simulink model "final_model"  (R2023b)
settings: Solver=VariableStepAuto  StartTime=0.0  StopTime=200  RelTol=1e-3
(part 1 of 3)
settings Model: Creator=Iustin  LastModifiedBy=Iustin

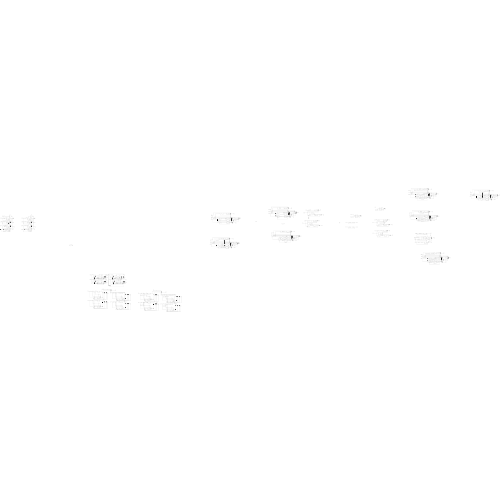
[thumbnail: Simulink's stored preview of the top-level diagram]
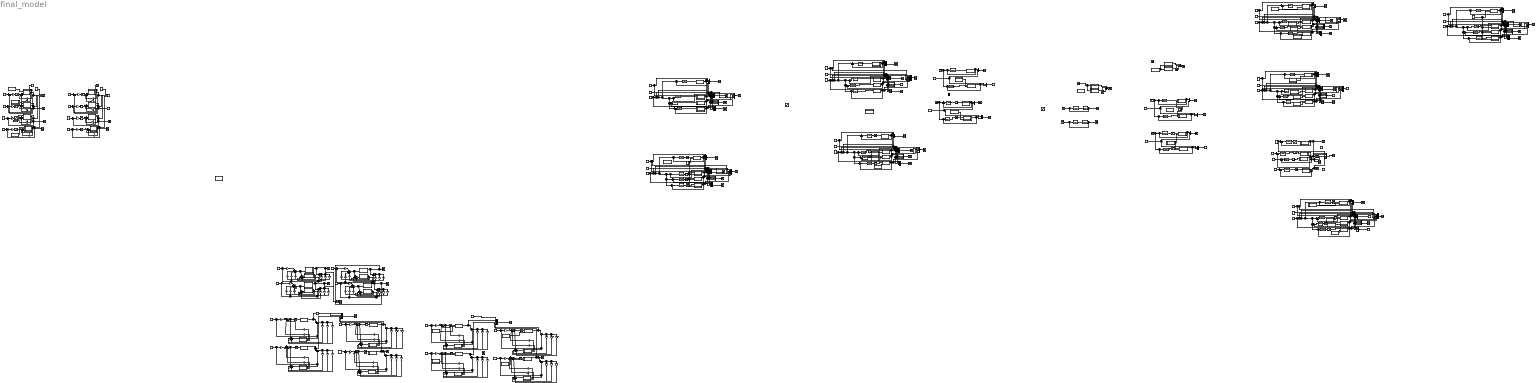
== system final_model ==
  "  G0 = 200" : Subsystem  mask{p1=0.005, p2=0.017, p3=0.00000808, n=0.175, V=120, Gb=80, G0=200}
  "  G0 = 4" : Subsystem  mask{p1=0.005, p2=0.017, p3=0.00000808, n=0.175, V=120, Gb=80, G0=200}
  " 100.1g" : Subsystem  mask{Gb=80, V=120, p1=0.032, p2=0.019, p3=0.00000987, n=0.208, G0=100}
  " 100.1g1" : Subsystem  mask{Gb=80, V=120, p1=0.032, p2=0.019, p3=0.00000987, n=0.208, G0=300}
  " G0 = 10" : Subsystem  mask{p1=0.005, p2=0.017, p3=0.00000808, n=0.175, V=120, Gb=80, G0=150}
  " G0 = 11" : Subsystem  mask{p1=0.005, p2=0.017, p3=0.00000808, n=0.175, V=120, Gb=80, G0=250}
  " G0 = 12" : Subsystem  mask{p1=0.005, p2=0.017, p3=0.00000808, n=0.175, V=120, Gb=80, G0=300}
  " G0 = 150" : Subsystem  mask{p1=0.005, p2=0.017, p3=0.00000808, n=0.175, V=120, Gb=80, G0=150}
  " G0 = 250" : Subsystem  mask{p1=0.005, p2=0.017, p3=0.00000808, n=0.175, V=120, Gb=80, G0=250}
  " G0 = 300" : Subsystem  mask{p1=0.005, p2=0.017, p3=0.00000808, n=0.175, V=120, Gb=80, G0=300}
  " Proces" : TransferFcn  Numerator=[-0.1741]  Denominator=[32320 6542 160.7 1]
  " Proces liniar" : Subsystem  mask{p1=0.005, p2=0.017, p3=0.00000808, n=0.175, V=120, Gb=80, G0=350, Xb=0.0054}
  " Proces liniar1" : Subsystem  mask{p1=0.005, p2=0.017, p3=0.00000808, n=0.175, V=120, Gb=80, G0=350, Xb=0.0054}
  " Proces liniar10" : Subsystem  mask{p1=0.005, p2=0.017, p3=0.00000808, n=0.175, V=120, Gb=80, G0=150, Xb=0.0054}
  " Proces liniar11" : Subsystem  mask{p1=0.005, p2=0.017, p3=0.00000808, n=0.175, V=120, Gb=80, G0=200, Xb=0.0054}
  " Proces liniar12" : Subsystem  mask{p1=0.005, p2=0.017, p3=0.00000808, n=0.175, V=120, Gb=80, G0=250, Xb=0.0054}
  " Proces liniar13" : Subsystem  mask{p1=0.005, p2=0.017, p3=0.00000808, n=0.175, V=120, Gb=80, G0=300, Xb=0.0054}
  " Proces liniar14" : Subsystem  mask{p1=0.005, p2=0.017, p3=0.00000808, n=0.175, V=120, Gb=80, G0=150, Xb=0.0054}
  " Proces liniar15" : Subsystem  mask{p1=0.005, p2=0.017, p3=0.00000808, n=0.175, V=120, Gb=80, G0=200, Xb=0.0054}
  " Proces liniar16" : Subsystem  mask{p1=0.005, p2=0.017, p3=0.00000808, n=0.175, V=120, Gb=80, G0=250, Xb=0.0054}
  " Proces liniar17" : Subsystem  mask{p1=0.005, p2=0.017, p3=0.00000808, n=0.175, V=120, Gb=80, G0=300, Xb=0.0054}
  " Proces liniar18" : Subsystem  mask{p1=0.005, p2=0.017, p3=0.00000808, n=0.175, V=120, Gb=80, G0=150, Xb=0.0054}
  " Proces liniar19" : Subsystem  mask{p1=0.005, p2=0.017, p3=0.00000808, n=0.175, V=120, Gb=80, G0=150, Xb=0.0054}
  " Proces liniar2" : Subsystem  mask{p1=0.005, p2=0.017, p3=0.00000808, n=0.175, V=120, Gb=80, G0=150, Xb=0.0054}
  " Proces liniar20" : Subsystem  mask{p1=0.005, p2=0.017, p3=0.00000808, n=0.175, V=120, Gb=80, G0=150, Xb=0.0054}
  " Proces liniar21" : Subsystem  mask{p1=0.005, p2=0.017, p3=0.00000808, n=0.175, V=120, Gb=80, G0=150, Xb=0.0054}
  " Proces liniar22" : Subsystem  mask{p1=0.005, p2=0.017, p3=0.00000808, n=0.175, V=120, Gb=80, G0=100, Xb=0.0054}
  " Proces liniar23" : Subsystem  mask{p1=0.005, p2=0.017, p3=0.00000808, n=0.175, V=120, Gb=80, G0=100, Xb=0.0054}
  " Proces liniar24" : Subsystem  mask{p1=0.005, p2=0.017, p3=0.00000808, n=0.175, V=120, Gb=80, G0=100, Xb=0.0054}
  " Proces liniar25" : Subsystem  mask{p1=0.005, p2=0.017, p3=0.00000808, n=0.175, V=120, Gb=80, G0=100, Xb=0.0054}
  " Proces liniar26" : Subsystem  mask{p1=0.005, p2=0.017, p3=0.00000808, n=0.175, V=120, Gb=80, G0=100, Xb=0.0054}
  " Proces liniar27" : Subsystem  mask{p1=0.005, p2=0.017, p3=0.00000808, n=0.175, V=120, Gb=80, G0=100, Xb=0.0054}
  " Proces liniar28" : Subsystem  mask{p1=0.005, p2=0.017, p3=0.00000808, n=0.175, V=120, Gb=80, G0=100, Xb=0.0054}
  " Proces liniar29" : Subsystem  mask{p1=0.005, p2=0.017, p3=0.00000808, n=0.175, V=120, Gb=80, G0=100, Xb=0.0054}
  " Proces liniar3" : Subsystem  mask{p1=0.005, p2=0.017, p3=0.00000808, n=0.175, V=120, Gb=80, G0=150, Xb=0.0054}
  " Proces liniar30" : Subsystem  mask{p1=0.005, p2=0.017, p3=0.00000808, n=0.175, V=120, Gb=80, G0=100, Xb=0.0054}
  " Proces liniar4" : Subsystem  mask{p1=0.005, p2=0.017, p3=0.00000808, n=0.175, V=120, Gb=80, G0=150, Xb=0.0054}
  " Proces liniar5" : Subsystem  mask{p1=0.005, p2=0.017, p3=0.00000808, n=0.175, V=120, Gb=80, G0=150, Xb=0.0054}
  " Proces liniar6" : Subsystem  mask{p1=0.005, p2=0.017, p3=0.00000808, n=0.175, V=120, Gb=80, G0=150, Xb=0.0054}
  " Proces liniar7" : Subsystem  mask{p1=0.005, p2=0.017, p3=0.00000808, n=0.175, V=120, Gb=80, G0=200, Xb=0.0054}
  " Proces liniar8" : Subsystem  mask{p1=0.005, p2=0.017, p3=0.00000808, n=0.175, V=120, Gb=80, G0=250, Xb=0.0054}
  " Proces liniar9" : Subsystem  mask{p1=0.005, p2=0.017, p3=0.00000808, n=0.175, V=120, Gb=80, G0=300, Xb=0.0054}
  " Proces neliniar" : Subsystem  mask{p1=0.005, p2=0.017, p3=0.00000808, n=0.175, V=120, Gb=80, G0=350}
  " Proces neliniar1" : Subsystem  mask{p1=0.005, p2=0.017, p3=0.00000808, n=0.175, V=120, Gb=80, G0=350}
  " Proces neliniar2" : Subsystem  mask{p1=0.005, p2=0.017, p3=0.00000808, n=0.175, V=120, Gb=80, G0=150}
  " Proces neliniar3" : Subsystem  mask{p1=0.005, p2=0.017, p3=0.00000808, n=0.175, V=120, Gb=80, G0=150}
  " Proces neliniar4" : Subsystem  mask{p1=0.005, p2=0.017, p3=0.00000808, n=0.175, V=120, Gb=80, G0=150}
  " Proces neliniar5" : Subsystem  mask{p1=0.005, p2=0.017, p3=0.00000808, n=0.175, V=120, Gb=80, G0=200}
  " Proces1" : TransferFcn  Numerator=[-0.1741]  Denominator=[32320 6542 160.7 1]
  " Regulator" : TransferFcn  Numerator=[-1454 -294.4 -7.231 -0.045]  Denominator=[171.2 34.28 1 0]
   Regulator plasar{,1..8,13..16} (13 alike) : TransferFcn  Numerator=[-1454 -294.4 -7.231 -0.045]  Denominator=[171.2 34.28 1 0]
  " Regulator plasare" : TransferFcn  Numerator=[-1454 -294.4 -7.231 -0.045]  Denominator=[171.2 34.28 1 0]
  " Regulator1" : TransferFcn  Numerator=[-1454 -294.4 -7.231 -0.045]  Denominator=[171.2 34.28 1 0]
   Regulator{2,4..6} (4 alike) : TransferFcn  Numerator=[-2843 -77.89 -0.5026]  Denominator=[0.5714 1 0]
  " Regulator3" : TransferFcn  Numerator=[-1454 -294.4 -7.231 -0.045]  Denominator=[171.2 34.28 1 0]
   RegulatorCMVK{,1..24} (25 alike) : TransferFcn  Numerator=[-2843 -77.89 -0.5026]  Denominator=[0.5714 1 0]
  10.1g : Subsystem  mask{Gb=80, V=120, p1=0.032, p2=0.019, p3=0.00000987, n=0.208, G0=100}
  10.1g1 : Subsystem  mask{Gb=80, V=120, p1=0.032, p2=0.019, p3=0.00000987, n=0.208, G0=150}
  1001g : Subsystem  mask{p1=0.005, p2=0.017, p3=0.00000808, n=0.175, V=120, Gb=80, G0=100}
  100g : Subsystem  mask{p1=0.005, p2=0.017, p3=0.00000808, n=0.175, V=120, Gb=80, G0=100}
  100g.1 : Subsystem  mask{p1=0.005, p2=0.017, p3=0.00000808, n=0.175, V=120, Gb=80, G0=100}
  10g : Subsystem  mask{p1=0.005, p2=0.017, p3=0.00000808, n=0.175, V=120, Gb=80, G0=100}
  10g.1 : Subsystem  mask{p1=0.005, p2=0.017, p3=0.00000808, n=0.175, V=120, Gb=80, G0=100}
  10g1 : Subsystem  mask{p1=0.005, p2=0.017, p3=0.00000808, n=0.175, V=120, Gb=80, G0=100}
  150gg : Subsystem  mask{p1=0.005, p2=0.017, p3=0.00000808, n=0.175, V=120, Gb=80, G0=150}
  200gg : Subsystem  mask{p1=0.005, p2=0.017, p3=0.00000808, n=0.175, V=120, Gb=80, G0=200}
  250gg : Subsystem  mask{p1=0.005, p2=0.017, p3=0.00000808, n=0.175, V=120, Gb=80, G0=250}
  300gg : Subsystem  mask{p1=0.005, p2=0.017, p3=0.00000808, n=0.175, V=120, Gb=80, G0=300}
  40.1g : Subsystem  mask{Gb=80, V=120, p1=0.032, p2=0.019, p3=0.00000987, n=0.208, G0=100}
  40.1g1 : Subsystem  mask{Gb=80, V=120, p1=0.032, p2=0.019, p3=0.00000987, n=0.208, G0=200}
  40g : Subsystem  mask{p1=0.005, p2=0.017, p3=0.00000808, n=0.175, V=120, Gb=80, G0=100}
  40g.1 : Subsystem  mask{p1=0.005, p2=0.017, p3=0.00000808, n=0.175, V=120, Gb=80, G0=100}
  40g1 : Subsystem  mask{p1=0.005, p2=0.017, p3=0.00000808, n=0.175, V=120, Gb=80, G0=100}
  70.1g : Subsystem  mask{Gb=80, V=120, p1=0.032, p2=0.019, p3=0.00000987, n=0.208, G0=100}
  70.1g1 : Subsystem  mask{Gb=80, V=120, p1=0.032, p2=0.019, p3=0.00000987, n=0.208, G0=250}
  70g : Subsystem  mask{p1=0.005, p2=0.017, p3=0.00000808, n=0.175, V=120, Gb=80, G0=100}
  70g.1 : Subsystem  mask{p1=0.005, p2=0.017, p3=0.00000808, n=0.175, V=120, Gb=80, G0=100}
  70g1 : Subsystem  mask{p1=0.005, p2=0.017, p3=0.00000808, n=0.175, V=120, Gb=80, G0=100}
  80 : Constant  Value=80
  Constant{,1..7,9,11..18,20..24,26..32} (29 alike) : Constant  Value=80
  Constant10 : Constant  Value=74
  Constant19 : Constant  Value=0
  Constant25 : Constant  Value=110
  Constant8 : Constant  Value=0
  DG 100g : Subsystem  mask{p1=0.005, p2=0.017, p3=0.00000808, n=0.175, V=120, Gb=80, G0=100}
  DG 10g : Subsystem  mask{p1=0.005, p2=0.017, p3=0.00000808, n=0.175, V=120, Gb=80, G0=100}
  DG 40g : Subsystem  mask{p1=0.005, p2=0.017, p3=0.00000808, n=0.175, V=120, Gb=80, G0=100}
  DG 70g : Subsystem  mask{p1=0.005, p2=0.017, p3=0.00000808, n=0.175, V=120, Gb=80, G0=100}
  K{1..3,10..13,25} (8 alike) : Gain  Gain=-10.1821
  K{4..6,14..15,17..18,36} (8 alike) : Gain  Gain=-1.4596e+05
  K{7..9,16,19..21,42} (8 alike) : Gain  Gain=0.0012
  K2.1 {,1..3} (4 alike) : Gain  Gain=-1.4472e+05
  K3.1 {,1..3} (4 alike) : Gain  Gain=-0.0018
  Ke1.{1..4} (4 alike) : Gain  Gain=-0.2134
  Ke2.{1..4} (4 alike) : Gain  Gain=0.0008
  Ke3.{1..4} (4 alike) : Gain  Gain=-8.4418
  Limita inferioara : Constant  Value=74
  Limita inferioara1 : Constant  Value=74
  Limita inferioara2 : Constant  Value=74
  Limita superioara : Constant  Value=110
  Limita superioara1 : Constant  Value=110
  Limita superioara2 : Constant  Value=110
  Maxim{1..5} (5 alike) : Constant  Value=110
  Minim{1..5} (5 alike) : Constant  Value=74
  Minim6 : Constant  Value=0
  Mux : Mux  Inputs=3
  Mux1 : Mux  Inputs=3
  Mux{3..10} (8 alike) : Mux  Inputs=2
  Mux11 : Mux  Inputs=7
  Mux{12..14,27,37,47,52..53} (8 alike) : Mux  Inputs=5
  Mux{15..26,28..31,33..36,38..41,43..46,48..51} (32 alike) : Mux
  Mux2 : Mux  Inputs=3
  Mux32 : Mux  Inputs=7
  Mux42 : Mux  Inputs=7
  Saturation : Saturate
  Saturation{1..12,14,18..22} (18 alike) : Saturate  UpperLimit=0  LowerLimit=-500
  Saturation{13,15..17,23..37} (19 alike) : Saturate  UpperLimit=500  LowerLimit=0
  Scope{,1..56,58..61,63..71,73..76} (74 alike) : Scope
  Scope57 : Scope  NumInputPorts=5
  Scope62 : Scope  NumInputPorts=5
  Scope72 : Scope  NumInputPorts=5
  Step{,1..9} (10 alike) : Step  SampleTime=0
  Sum{,1..46,48,50,52,54,57..58,62,64..65,68..70,73..74,77..78,81..82,85..86,89..90,93..94,97..98,101..102,104,106,108} (78 alike) : Sum  Inputs=|+-
  Sum{55..56,59..61,63,66..67,72,76,80,84,88,92,96,100} (16 alike) : Sum  Inputs=|++++
  Sum{47,49,51,53,103,105,107,109} (8 alike) : Sum  Inputs=|+++
  Sum{71,75,79,83,87,91,95,99} (8 alike) : Sum  Inputs=|+--
  Val. optima : Constant  Value=80
  Val. optima1 : Constant  Value=80
  Valoare optima{,1..7} (8 alike) : Constant  Value=80
  con : Constant  Value=80
  k{1,4,7,10,13..14,19,22} (8 alike) : Gain  Gain=-10.1821
  k1.1 {,1..3} (4 alike) : Gain  Gain=-45.1979
  k{2,5,8,11,15,17,20,23} (8 alike) : Gain  Gain=1.4596e+05
  k{3,6,9,12,16,18,21,24} (8 alike) : Gain  Gain=0.0012
  ke{1,4,7,10,13..14,19,22} (8 alike) : Gain  Gain=0.3304
  ke{2,5,8,11,15,17,20,23} (8 alike) : Gain  Gain=3.3886e-04
  ke{3,6,9,12,16,18,21,24} (8 alike) : Gain  Gain=0.1231
  kr.{1..4} (4 alike) : Gain  Gain=-9.1200e-04
  model liniar1 : Subsystem  mask{p1=0.032, p2=0.019, p3=0.00000987, V=120, Gb=80, Xb=0.0054, n=0.208, G0=150}
  model liniar2 : Subsystem  mask{p1=0.032, p2=0.019, p3=0.00000987, V=120, Gb=80, Xb=0.0054, n=0.208, G0=200}
  model liniar3 : Subsystem  mask{p1=0.032, p2=0.019, p3=0.00000987, V=120, Gb=80, Xb=0.0054, n=0.208, G0=250}
  model liniar4 : Subsystem  mask{p1=300, p2=0.019, p3=0.00000987, V=120, Gb=80, Xb=0.0054, n=0.208, G0=300}
  model_neliniar1 : Subsystem  mask{Gb=80, V=120, p1=0.032, p2=0.019, p3=0.00000987, n=0.208, G0=150}
  model_neliniar2 : Subsystem  mask{Gb=80, V=120, p1=0.032, p2=0.019, p3=0.00000987, n=0.208, G0=200}
  model_neliniar3 : Subsystem  mask{Gb=80, V=120, p1=0.032, p2=0.019, p3=0.00000987, n=0.208, G0=250}
  model_neliniar4 : Subsystem  mask{Gb=80, V=120, p1=0.032, p2=0.019, p3=0.00000987, n=0.208, G0=300}
  perturbatie1 : Subsystem  mask{Dg=100000, Ag=0.8, tg_max=40}
  perturbatie10 : Subsystem  mask{Dg=40*1000, Ag=0.8, tg_max=40}
  perturbatie11 : Subsystem  mask{Dg=100000, Ag=0.8, tg_max=40}
  perturbatie12 : Subsystem  mask{Dg=70*1000, Ag=0.8, tg_max=40}
  perturbatie13 : Subsystem  mask{Dg=100*1000, Ag=0.8, tg_max=40}
  perturbatie15 : Subsystem  mask{Dg=40*1000, Ag=0.8, tg_max=40}
  perturbatie16 : Subsystem  mask{Dg=70*1000, Ag=0.8, tg_max=40}
  perturbatie17 : Subsystem  mask{Dg=100*1000, Ag=0.8, tg_max=40}
  perturbatie18 : Subsystem  mask{Dg=10*1000, Ag=0.8, tg_max=40}
  perturbatie19 : Subsystem  mask{Dg=40, Ag=0.8, tg_max=40}
  perturbatie2 : Subsystem  mask{Dg=100000, Ag=0.8, tg_max=40}
  perturbatie20 : Subsystem  mask{Dg=70, Ag=0.8, tg_max=40}
  perturbatie21 : Subsystem  mask{Dg=100, Ag=0.8, tg_max=40}
  perturbatie22 : Subsystem  mask{Dg=10, Ag=0.8, tg_max=40}
  perturbatie23 : Subsystem  mask{Dg=40*1000, Ag=0.8, tg_max=40}
  perturbatie24 : Subsystem  mask{Dg=70*1000, Ag=0.8, tg_max=40}
  perturbatie25 : Subsystem  mask{Dg=100*1000, Ag=0.8, tg_max=40}
  perturbatie29 : Subsystem  mask{Dg=40*1000, Ag=0.8, tg_max=40}
  perturbatie3 : Subsystem  mask{Dg=10, Ag=0.8, tg_max=40}
  perturbatie30 : Subsystem  mask{Dg=70*1000, Ag=0.8, tg_max=40}
  perturbatie31 : Subsystem  mask{Dg=100*1000, Ag=0.8, tg_max=40}
  perturbatie36 : Subsystem  mask{Dg=10*1000, Ag=0.8, tg_max=40}
  perturbatie37 : Subsystem  mask{Dg=40*1000, Ag=0.8, tg_max=40}
  perturbatie38 : Subsystem  mask{Dg=70*1000, Ag=0.8, tg_max=40}
  perturbatie39 : Subsystem  mask{Dg=100*1000, Ag=0.8, tg_max=40}
  perturbatie4 : Subsystem  mask{Dg=10, Ag=0.8, tg_max=40}
  perturbatie5 : Subsystem  mask{Dg=10, Ag=0.8, tg_max=40}
  perturbatie6 : Subsystem  mask{Dg=30, Ag=0.8, tg_max=40}
  perturbatie7 : Subsystem  mask{Dg=40*1000, Ag=0.8, tg_max=40}
  perturbatie8 : Subsystem  mask{Dg=10*1000, Ag=0.8, tg_max=40}
  perturbatie9 : Subsystem  mask{Dg=10*1000, Ag=0.8, tg_max=40}
  wires:
  " Proces liniar"/1(" G(t)") -> Mux/1
  " Proces neliniar"/1(" G(t)") -> Mux/2
  Step/1 -> Mux/3
  Mux/1 -> Scope/1
  perturbatie1/1(p(t)) -> " Proces liniar"/2(p(t)), " Proces neliniar"/2(p(t))
  Mux1/1 -> Scope1/1
  Step2/1 -> Mux1/3
  " Proces neliniar1"/1(" G(t)") -> Mux1/2
  " Proces liniar1"/1(" G(t)") -> Mux1/1
  Step3/1 -> " Proces neliniar1"/1(" u(t)"), " Proces liniar1"/1(" u(t)")
  Sum/1 -> " Regulator"/1
  " Regulator"/1 -> " Proces"/1
  Step6/1 -> Sum2/1, Sum1/1
  Sum1/1 -> " Regulator1"/1
  " Regulator1"/1 -> Saturation2/1
  " Proces neliniar2"/1(" G(t)") -> Sum2/2, Mux3/1
  " Proces liniar2"/1(" G(t)") -> Mux4/1, Sum1/2
  Sum2/1 -> " Regulator plasare"/1
  " Regulator plasare"/1 -> Saturation1/1
  Saturation1/1 -> " Proces neliniar2"/1(" u(t)")
  Mux3/1 -> Scope4/1
  Constant/1 -> Mux4/2, Mux3/2
  Mux4/1 -> Scope3/1
  Saturation2/1 -> " Proces liniar2"/1(" u(t)")
  " Proces"/1 -> Scope2/1, Sum/2
  " Regulator3"/1 -> " Proces liniar3"/1(" u(t)")
  " Proces neliniar3"/1(" G(t)") -> Sum4/2, Mux6/1
  Mux6/1 -> Scope6/1
  Mux7/1 -> Scope5/1
  " Regulator plasar"/1 -> " Proces neliniar3"/1(" u(t)")
  Constant3/1 -> Mux7/2, Mux6/2
  Sum3/1 -> " Regulator3"/1
  " Proces liniar3"/1(" G(t)") -> Mux7/1, Sum3/2
  Step5/1 -> Sum4/1, Sum3/1
  perturbatie4/1(p(t)) -> " Proces neliniar3"/2(p(t))
  Sum4/1 -> " Regulator plasar"/1
  Step4/1 -> Sum/1
  Sum5/1 -> " Regulator5"/1
  " Regulator5"/1 -> " Proces1"/1
  " Proces1"/1 -> Scope7/1, Sum5/2
  Step7/1 -> Sum5/1
  " Proces liniar4"/1(" G(t)") -> Mux8/1, Sum6/2
  Constant1/1 -> Mux8/2, Mux5/2
  " Regulator4"/1 -> " Proces liniar4"/1(" u(t)")
  " Regulator2"/1 -> " Proces neliniar4"/1(" u(t)")
  Mux8/1 -> Scope8/1
  Mux5/1 -> Scope9/1
  Step8/1 -> Sum7/1, Sum6/1
  " Proces neliniar4"/1(" G(t)") -> Sum7/2, Mux5/1
  Sum7/1 -> " Regulator2"/1
  Sum6/1 -> " Regulator4"/1
  " Regulator6"/1 -> Saturation5/1
  " Proces neliniar5"/1(" G(t)") -> Sum9/2, Mux9/1
  Mux9/1 -> Scope11/1
  Saturation5/1 -> " Proces neliniar5"/1(" u(t)")
  Saturation6/1 -> " Proces liniar5"/1(" u(t)")
  Step9/1 -> Sum9/1, Sum8/1
  Mux10/1 -> Scope10/1
  Constant2/1 -> Mux10/2, Mux9/2
  Sum8/1 -> " RegulatorCMVK"/1
  " RegulatorCMVK"/1 -> Saturation6/1
  " Proces liniar5"/1(" G(t)") -> Mux10/1, Sum8/2
  Sum9/1 -> " Regulator6"/1
  perturbatie6/1(p(t)) -> " Proces neliniar5"/2(p(t)), " Proces liniar5"/2(p(t))
  perturbatie3/1(p(t)) -> " Proces neliniar2"/2(p(t))
  Sum10/1 -> " Regulator plasar1"/1
  Sum11/1 -> " Regulator plasar2"/1
  Sum12/1 -> " Regulator plasar3"/1
  Sum13/1 -> " Regulator plasar4"/1
  Mux11/1 -> Scope16/1
  Constant19/1 -> " Proces neliniar4"/2(p(t)), " Proces liniar4"/2(p(t))
  Sum22/1 -> " RegulatorCMVK5"/1
  Sum23/1 -> " RegulatorCMVK6"/1
  Constant23/1 -> Sum24/1
  Constant24/1 -> Sum25/1
  10g/1(" G(t)") -> Sum22/2, Mux14/1, Scope27/1
  " RegulatorCMVK5"/1 -> Saturation9/1
  Mux14/1 -> Scope31/1
  80/1 -> Mux14/5, Sum22/1
  " RegulatorCMVK6"/1 -> Saturation10/1
  70g/1(" G(t)") -> Scope29/1, Mux14/3, Sum24/2
  Sum24/1 -> " RegulatorCMVK7"/1
  100g/1(" G(t)") -> Mux14/4, Scope28/1, Sum25/2
  40g/1(" G(t)") -> Mux14/2, Scope30/1, Sum23/2
  con/1 -> Sum23/1
  Sum25/1 -> " RegulatorCMVK8"/1
  " RegulatorCMVK7"/1 -> Saturation11/1
  Saturation9/1 -> 10g/1(" u(t)")
  Saturation10/1 -> 40g/1(" u(t)")
  Saturation11/1 -> 70g/1(" u(t)")
  " RegulatorCMVK8"/1 -> Saturation12/1
  Saturation12/1 -> 100g/1(" u(t)")
  Mux16/1 -> Scope12/1
  Valoare optima/1 -> Mux19/4, Mux18/4, Mux17/4, Mux11/5, Mux16/4, Sum10/1, Sum13/1, Sum12/1, Sum11/1
  " G0 = 300"/1(" G(t)") -> Mux11/4, Mux19/1, Sum13/2
  Mux19/1 -> Scope13/1
  "  G0 = 200"/1(" G(t)") -> Mux11/2, Mux17/1, Sum11/2
  Mux17/1 -> Scope15/1
  Mux18/1 -> Scope14/1
  " G0 = 150"/1(" G(t)") -> Sum10/2, Mux11/1, Mux16/1
  Limita inferioara/1 -> Mux19/2, Mux18/2, Mux17/2, Mux11/7, Mux16/2
  Limita superioara/1 -> Mux11/6, Mux19/3, Mux18/3, Mux17/3, Mux16/3
  " G0 = 250"/1(" G(t)") -> Mux11/3, Mux18/1, Sum12/2
  DG 40g/1(" G(t)") -> Mux12/2, Mux21/1, Sum15/2
  DG 70g/1(" G(t)") -> Mux12/3, Mux22/1, Sum16/2
  Minim1/1 -> Mux23/2, Mux22/2, Mux21/2, Mux20/2
  Mux22/1 -> Scope19/1
  Mux21/1 -> Scope20/1
  Mux20/1 -> Scope17/1
  DG 10g/1(" G(t)") -> Sum14/2, Mux12/1, Mux20/1
  Maxim1/1 -> Mux20/3, Mux23/3, Mux22/3, Mux21/3
  Valoare optima1/1 -> Mux23/4, Mux22/4, Mux21/4, Mux12/5, Mux20/4, Sum14/1, Sum17/1, Sum16/1, Sum15/1
  Mux12/1 -> Scope21/1
  Sum16/1 -> " Regulator plasar7"/1
  DG 100g/1(" G(t)") -> Mux12/4, Mux23/1, Sum17/2
  Sum15/1 -> " Regulator plasar6"/1
  Sum17/1 -> " Regulator plasar8"/1
  Sum14/1 -> " Regulator plasar5"/1
  Mux23/1 -> Scope18/1
  " Regulator plasar5"/1 -> Saturation22/1
  " Regulator plasar6"/1 -> Saturation4/1
  " Regulator plasar7"/1 -> Saturation7/1
  40g1/1(" G(t)") -> Mux13/2, Mux24/1, Sum19/2
  " RegulatorCMVK2"/1 -> 40g1/1(" u(t)")
  70g1/1(" G(t)") -> Mux13/3, Mux25/1, Sum20/2
  Minim2/1 -> Mux26/2, Mux25/2, Mux24/2, Mux15/2
  Mux25/1 -> Scope24/1
  " RegulatorCMVK3"/1 -> 70g1/1(" u(t)")
  Mux24/1 -> Scope25/1
  Mux15/1 -> Scope22/1
  " RegulatorCMVK4"/1 -> 1001g/1(" u(t)")
  10g1/1(" G(t)") -> Sum18/2, Mux13/1, Mux15/1
  Maxim2/1 -> Mux15/3, Mux26/3, Mux25/3, Mux24/3
  Valoare optima2/1 -> Mux26/4, Mux25/4, Mux24/4, Mux13/5, Mux15/4, Sum18/1, Sum21/1, Sum20/1, Sum19/1
  Mux13/1 -> Scope26/1
  Sum20/1 -> " RegulatorCMVK3"/1
  1001g/1(" G(t)") -> Mux13/4, Mux26/1, Sum21/2
  Sum19/1 -> " RegulatorCMVK2"/1
  Sum21/1 -> " RegulatorCMVK4"/1
  Sum18/1 -> " RegulatorCMVK1"/1
  Mux26/1 -> Scope23/1
  " RegulatorCMVK1"/1 -> 10g1/1(" u(t)")
  " Proces liniar6"/1(" G(t)") -> Sum26/2, Mux27/1, Mux28/1
  " RegulatorCMVK20"/1 -> " Proces liniar9"/1(" u(t)")
  Mux31/1 -> Scope33/1
  Maxim3/1 -> Mux31/3, Mux30/3, Mux29/3, Mux28/3
  Minim3/1 -> Mux31/2, Mux30/2, Mux29/2, Mux28/2
  Sum27/1 -> " RegulatorCMVK18"/1
  Mux30/1 -> Scope34/1
  " RegulatorCMVK19"/1 -> " Proces liniar8"/1(" u(t)")
  " Proces liniar7"/1(" G(t)") -> Mux27/2, Mux29/1, Sum27/2
  Valoare optima3/1 -> Mux31/4, Mux30/4, Mux29/4, Mux27/5, Mux28/4, Sum26/1, Sum29/1, Sum28/1, Sum27/1
  " Proces liniar9"/1(" G(t)") -> Mux27/4, Mux31/1, Sum29/2
  Mux28/1 -> Scope32/1
  Mux27/1 -> Scope36/1
  " RegulatorCMVK17"/1 -> " Proces liniar6"/1(" u(t)")
  Sum29/1 -> " RegulatorCMVK20"/1
  " Proces liniar8"/1(" G(t)") -> Mux27/3, Mux30/1, Sum28/2
  Sum28/1 -> " RegulatorCMVK19"/1
  " RegulatorCMVK18"/1 -> " Proces liniar7"/1(" u(t)")
  Mux29/1 -> Scope35/1
  Sum26/1 -> " RegulatorCMVK17"/1
  Sum30/1 -> " Regulator plasar16"/1
  " Regulator plasar13"/1 -> Saturation15/1
  " Proces liniar13"/1(" G(t)") -> Mux32/4, Mux36/1, Sum33/2
  Sum32/1 -> " Regulator plasar14"/1
  " Proces liniar11"/1(" G(t)") -> Mux32/2, Mux34/1, Sum31/2
  " Regulator plasar16"/1 -> Saturation14/1
  Mux34/1 -> Scope40/1
  Constant8/1 -> " Proces liniar10"/2(p(t)), " Proces liniar11"/2(p(t)), " Proces liniar13"/2(p(t)), " Proces liniar12"/2(p(t))
  Sum33/1 -> " Regulator plasar15"/1
  " Proces liniar12"/1(" G(t)") -> Mux32/3, Mux35/1, Sum32/2
  Mux32/1 -> Scope41/1
  Mux33/1 -> Scope37/1
  " Regulator plasar14"/1 -> Saturation16/1
  Sum31/1 -> " Regulator plasar13"/1
  Mux35/1 -> Scope39/1
  Maxim4/1 -> Mux32/7, Mux36/3, Mux35/3, Mux34/3, Mux33/3
  Minim4/1 -> Mux36/2, Mux35/2, Mux34/2, Mux32/6, Mux33/2
  " Regulator plasar15"/1 -> Saturation17/1
  Valoare optima4/1 -> Mux36/4, Mux35/4, Mux34/4, Mux32/5, Mux33/4, Sum30/1, Sum33/1, Sum32/1, Sum31/1
  Mux36/1 -> Scope38/1
  " Proces liniar10"/1(" G(t)") -> Sum30/2, Mux32/1, Mux33/1
  Saturation14/1 -> " Proces liniar10"/1(" u(t)")
  Saturation15/1 -> " Proces liniar11"/1(" u(t)")
  Saturation16/1 -> " Proces liniar12"/1(" u(t)")
  Saturation17/1 -> " Proces liniar13"/1(" u(t)")
  perturbatie18/1(p(t)) -> " Proces liniar18"/2(p(t))
  perturbatie15/1(p(t)) -> " Proces liniar19"/2(p(t))
  perturbatie16/1(p(t)) -> " Proces liniar20"/2(p(t))
  Mux41/1 -> Scope43/1
  Limita superioara1/1 -> Mux41/3, Mux40/3, Mux39/3, Mux38/3
  " Proces liniar18"/1(" G(t)") -> Sum34/2, Mux37/1, Mux38/1
  " RegulatorCMVK9"/1 -> " Proces liniar18"/1(" u(t)")
  Mux40/1 -> Scope44/1
  " Proces liniar20"/1(" G(t)") -> Mux37/3, Mux40/1, Sum36/2
  Limita inferioara1/1 -> Mux41/2, Mux40/2, Mux39/2, Mux38/2
  Mux39/1 -> Scope45/1
  " Proces liniar19"/1(" G(t)") -> Mux37/2, Mux39/1, Sum35/2
  Mux38/1 -> Scope42/1
  Valoare optima5/1 -> Mux41/4, Mux40/4, Mux39/4, Mux37/5, Mux38/4, Sum34/1, Sum37/1, Sum36/1, Sum35/1
  Sum37/1 -> " RegulatorCMVK11"/1
  Mux37/1 -> Scope46/1
  Sum34/1 -> " RegulatorCMVK9"/1
  Sum36/1 -> " RegulatorCMVK12"/1
  Sum35/1 -> " RegulatorCMVK10"/1
  " RegulatorCMVK10"/1 -> " Proces liniar19"/1(" u(t)")
  " RegulatorCMVK12"/1 -> " Proces liniar20"/1(" u(t)")
  " RegulatorCMVK13"/1 -> Saturation19/1
  Sum41/1 -> " RegulatorCMVK14"/1
  Sum39/1 -> " RegulatorCMVK13"/1
  " G0 = 10"/1(" G(t)") -> Sum38/2, Mux42/1, Mux43/1
  Sum38/1 -> " RegulatorCMVK16"/1
  " RegulatorCMVK16"/1 -> Saturation18/1
  Limita inferioara2/1 -> Mux46/2, Mux45/2, Mux44/2, Mux42/7, Mux43/2
  "  G0 = 4"/1(" G(t)") -> Mux42/2, Mux44/1, Sum39/2
  Mux43/1 -> Scope47/1
  perturbatie19/1(p(t)) -> "  G0 = 4"/2(p(t))
  perturbatie22/1(p(t)) -> " G0 = 10"/2(p(t))
  Limita superioara2/1 -> Mux42/6, Mux46/3, Mux45/3, Mux44/3, Mux43/3
  Mux46/1 -> Scope48/1
  Mux42/1 -> Scope51/1
  Valoare optima6/1 -> Mux46/4, Mux45/4, Mux44/4, Mux42/5, Mux43/4, Sum38/1, Sum41/1, Sum40/1, Sum39/1
  " G0 = 12"/1(" G(t)") -> Mux42/4, Mux46/1, Sum41/2
  Mux44/1 -> Scope50/1
  perturbatie20/1(p(t)) -> " G0 = 11"/2(p(t))
  perturbatie21/1(p(t)) -> " G0 = 12"/2(p(t))
  " G0 = 11"/1(" G(t)") -> Mux42/3, Mux45/1, Sum40/2
  " RegulatorCMVK14"/1 -> Saturation21/1
  Sum40/1 -> " RegulatorCMVK15"/1
  Mux45/1 -> Scope49/1
  Saturation18/1 -> " G0 = 10"/1(" u(t)")
  Saturation19/1 -> "  G0 = 4"/1(" u(t)")
  " RegulatorCMVK15"/1 -> Saturation20/1
  Saturation20/1 -> " G0 = 11"/1(" u(t)")
  Saturation21/1 -> " G0 = 12"/1(" u(t)")
  " Regulator plasar1"/1 -> " G0 = 150"/1(" u(t)")
  " Regulator plasar2"/1 -> "  G0 = 200"/1(" u(t)")
  " Regulator plasar3"/1 -> " G0 = 250"/1(" u(t)")
  " Regulator plasar4"/1 -> " G0 = 300"/1(" u(t)")
  Saturation22/1 -> DG 10g/1(" u(t)")
  Saturation4/1 -> DG 40g/1(" u(t)")
  Saturation7/1 -> DG 70g/1(" u(t)")
  " Regulator plasar8"/1 -> Saturation8/1
  Saturation8/1 -> DG 100g/1(" u(t)")
  perturbatie23/1(p(t)) -> DG 40g/2(p(t))
  perturbatie24/1(p(t)) -> DG 70g/2(p(t))
  perturbatie25/1(p(t)) -> DG 100g/2(p(t))
  perturbatie9/1(p(t)) -> 10g1/2(p(t))
  perturbatie29/1(p(t)) -> 40g1/2(p(t))
  perturbatie30/1(p(t)) -> 70g1/2(p(t))
  perturbatie31/1(p(t)) -> 1001g/2(p(t))
  Sum43/1 -> " RegulatorCMVK22"/1
  " RegulatorCMVK22"/1 -> " Proces liniar15"/1(" u(t)")
  Sum44/1 -> " RegulatorCMVK23"/1
  Sum42/1 -> " RegulatorCMVK21"/1
  Minim5/1 -> Mux51/2, Mux50/2, Mux49/2, Mux48/2
  Mux48/1 -> Scope52/1
  " RegulatorCMVK24"/1 -> " Proces liniar17"/1(" u(t)")
  Maxim5/1 -> Mux51/3, Mux50/3, Mux49/3, Mux48/3
  " Proces liniar15"/1(" G(t)") -> Mux47/2, Mux49/1, Sum43/2
  Mux50/1 -> Scope54/1
  " Proces liniar16"/1(" G(t)") -> Mux47/3, Mux50/1, Sum44/2
  Mux47/1 -> Scope56/1
  Valoare optima7/1 -> Mux51/4, Mux50/4, Mux49/4, Mux47/5, Mux48/4, Sum42/1, Sum45/1, Sum44/1, Sum43/1
  " Proces liniar17"/1(" G(t)") -> Mux47/4, Mux51/1, Sum45/2
  " Proces liniar14"/1(" G(t)") -> Sum42/2, Mux47/1, Mux48/1
  " RegulatorCMVK21"/1 -> " Proces liniar14"/1(" u(t)")
  Mux51/1 -> Scope53/1
  Mux49/1 -> Scope55/1
  Sum45/1 -> " RegulatorCMVK24"/1
  " RegulatorCMVK23"/1 -> " Proces liniar16"/1(" u(t)")
  Minim6/1 -> " Proces liniar15"/2(p(t)), " Proces liniar16"/2(p(t)), " Proces liniar17"/2(p(t)), " Proces liniar14"/2(p(t))
  " RegulatorCMVK11"/1 -> " Proces liniar21"/1(" u(t)")
  perturbatie17/1(p(t)) -> " Proces liniar21"/2(p(t))
  " Proces liniar21"/1(" G(t)") -> Sum37/2, Mux37/4, Mux41/1
  Val. optima/1 -> Scope57/1
  " 100.1g"/1(G(t)) -> Scope61/1, Scope57/5, Sum52/2
  40.1g/1(G(t)) -> Scope57/3, Scope59/1, Sum48/2
  Sum48/1 -> K1/1
  Sum50/1 -> K2/1
  70.1g/2(X(t)) -> K5/1
  10.1g/3(I(t)) -> K42/1
  Constant12/1 -> Sum50/1
  10.1g/1(G(t)) -> Sum46/2, Scope57/2, Scope58/1
  40.1g/3(I(t)) -> K7/1
  " 100.1g"/3(I(t)) -> K9/1
  K8/1 -> Sum51/3
  K5/1 -> Sum51/2
  K7/1 -> Sum49/3
  Sum53/1 -> " 100.1g"/2(u(t))
  40.1g/2(X(t)) -> K4/1
  K6/1 -> Sum53/2
  K4/1 -> Sum49/2
  70.1g/3(I(t)) -> K8/1
  70.1g/1(G(t)) -> Scope57/4, Scope60/1, Sum50/2
  " 100.1g"/2(X(t)) -> K6/1
  Sum52/1 -> K3/1
  Constant11/1 -> Sum48/1
  Constant4/1 -> Sum46/1
  Constant13/1 -> Sum52/1
  Sum49/1 -> 40.1g/2(u(t))
  K9/1 -> Sum53/3
  Sum46/1 -> K25/1
  Sum51/1 -> 70.1g/2(u(t))
  K42/1 -> Sum47/3
  10.1g/2(X(t)) -> K36/1
  K36/1 -> Sum47/2
  Sum47/1 -> 10.1g/2(u(t))
  perturbatie36/1(p(t)) -> 10.1g/1(p(t))
  perturbatie37/1(p(t)) -> 40.1g/1(p(t))
  perturbatie38/1(p(t)) -> 70.1g/1(p(t))
  perturbatie39/1(p(t)) -> " 100.1g"/1(p(t))
  K25/1 -> Saturation23/1
  Saturation23/1 -> Sum47/1
  K1/1 -> Saturation13/1
  Saturation13/1 -> Sum49/1
  K2/1 -> Saturation24/1
  Saturation24/1 -> Sum51/1
  K3/1 -> Saturation25/1
  Saturation25/1 -> Sum53/1
  model liniar3/1(G(t)) -> K3.1 2/1
  K3.1 3/1 -> Sum55/4
  Ke2.4/1 -> Sum56/3
  Ke3.1/1 -> Sum61/2
  Sum60/1 -> model_neliniar1/2(u(t)), Sum61/1
  Sum59/1 -> Sum63/1, model_neliniar2/2(u(t))
  kr.4/1 -> Sum55/1
  Constant9/1 -> Sum65/1
  Sum56/1 -> model liniar4/2(u(t))
  K2.1 3/1 -> Sum55/2
  Ke2.1/1 -> Sum61/3
  Sum57/1 -> Ke1.4/1, Ke2.4/1, Ke3.4/1
  model_neliniar3/1(G(t)) -> Sum68/1, Scope62/4, Scope64/1
  Sum62/1 -> Ke1.1/1, Ke2.1/1, Ke3.1/1
  model liniar3/2(X(t)) -> K2.1 2/1
  Sum64/1 -> Ke1.2/1, Ke2.2/1, Ke3.2/1
  Sum63/1 -> model liniar2/2(u(t))
  model liniar2/2(X(t)) -> K2.1 1/1
  Ke3.2/1 -> Sum63/2
  model liniar1/3(I(t)) -> Sum62/2, Sum58/2, "k1.1 "/1
  "K3.1 "/1 -> Sum60/4
  kr.2/1 -> Sum59/1
  Ke1.2/1 -> Sum63/4
  k1.1 1/1 -> Sum59/3
  Sum54/1 -> kr.2/1
  model liniar2/1(G(t)) -> K3.1 1/1
  Constant5/1 -> Scope62/1
  Sum61/1 -> model liniar1/2(u(t))
  Sum58/1 -> kr.1/1
  "K2.1 "/1 -> Sum60/2
  Ke1.1/1 -> Sum61/4
  kr.3/1 -> Sum66/1
  Ke2.2/1 -> Sum63/3
  K2.1 1/1 -> Sum59/2
  model liniar4/1(G(t)) -> K3.1 3/1
  model liniar4/2(X(t)) -> K2.1 3/1
  K3.1 2/1 -> Sum66/4
  k1.1 2/1 -> Sum66/3
  model_neliniar4/1(G(t)) -> Sum57/1, Scope65/1, Scope62/5
  Ke1.3/1 -> Sum67/4
  kr.1/1 -> Sum60/1
  model liniar1/1(G(t)) -> "K3.1 "/1
  k1.1 3/1 -> Sum55/3
  Sum68/1 -> Ke1.3/1, Ke2.3/1, Ke3.3/1
  Ke3.4/1 -> Sum56/2
  Sum67/1 -> model liniar3/2(u(t))
  model_neliniar1/1(G(t)) -> Sum62/1, Scope62/2, Scope66/1
  model_neliniar2/1(G(t)) -> Sum64/1, Scope62/3, Scope63/1
  model liniar3/3(I(t)) -> Sum68/2, Sum65/2, k1.1 2/1
  Constant6/1 -> Sum58/1
  Ke1.4/1 -> Sum56/4
  Ke3.3/1 -> Sum67/2
  model liniar2/3(I(t)) -> Sum64/2, Sum54/2, k1.1 1/1
  model liniar1/2(X(t)) -> "K2.1 "/1
  "k1.1 "/1 -> Sum60/3
  model liniar4/3(I(t)) -> Sum57/2, Sum69/2, k1.1 3/1
  Ke2.3/1 -> Sum67/3
  Constant7/1 -> Sum54/1
  Sum66/1 -> model_neliniar3/2(u(t)), Sum67/1
  Constant14/1 -> Sum69/1
  Sum69/1 -> kr.4/1
  Sum65/1 -> kr.3/1
  Sum55/1 -> model_neliniar4/2(u(t)), Sum56/1
  K3.1 1/1 -> Sum59/4
  K2.1 2/1 -> Sum66/2
  Constant15/1 -> Sum70/1
  Sum70/1 -> k1/1
  k1/1 -> Sum71/1
  Sum71/1 -> Saturation26/1, Sum72/1
  Sum72/1 -> " Proces liniar23"/1(" u(t)")
  150gg/1(" G(t)") -> Mux52/1, Sum73/1
  Sum73/1 -> ke1/1, ke2/1, ke3/1
  ke1/1 -> Sum72/2
  ke2/1 -> Sum72/3
  ke3/1 -> Sum72/4
  " Proces liniar23"/3(I(t)) -> k3/1
  " Proces liniar23"/2(X(t)) -> k2/1
  " Proces liniar23"/1(" G(t)") -> Sum70/2, Sum73/2
  k2/1 -> Sum71/3
  k3/1 -> Sum71/2
  Mux52/1 -> Scope67/1
  Constant16/1 -> Mux52/2
  Saturation26/1 -> 150gg/1(" u(t)")
  200gg/1(" G(t)") -> Mux52/3, Sum77/1
  k4/1 -> Sum75/1
  Saturation27/1 -> 200gg/1(" u(t)")
  ke5/1 -> Sum76/3
  Sum77/1 -> ke4/1, ke5/1, ke6/1
  " Proces liniar24"/3(I(t)) -> k6/1
  k5/1 -> Sum75/2
  " Proces liniar24"/2(X(t)) -> k5/1
  Constant17/1 -> Sum74/1
  Sum76/1 -> " Proces liniar24"/1(" u(t)")
  ke4/1 -> Sum76/2
  ke6/1 -> Sum76/4
  Sum74/1 -> k4/1
  Sum75/1 -> Saturation27/1, Sum76/1
  " Proces liniar24"/1(" G(t)") -> Sum74/2, Sum77/2
  k6/1 -> Sum75/3
  250gg/1(" G(t)") -> Mux52/4, Sum81/1
  k7/1 -> Sum79/1
  Saturation28/1 -> 250gg/1(" u(t)")
  ke8/1 -> Sum80/3
  Sum81/1 -> ke7/1, ke8/1, ke9/1
  " Proces liniar25"/3(I(t)) -> k9/1
  k8/1 -> Sum79/2
  " Proces liniar25"/2(X(t)) -> k8/1
  Constant20/1 -> Sum78/1
  Sum80/1 -> " Proces liniar25"/1(" u(t)")
  ke7/1 -> Sum80/2
  ke9/1 -> Sum80/4
  Sum78/1 -> k7/1
  Sum79/1 -> Saturation28/1, Sum80/1
  " Proces liniar25"/1(" G(t)") -> Sum78/2, Sum81/2
  k9/1 -> Sum79/3
  k10/1 -> Sum83/1
  Saturation29/1 -> 300gg/1(" u(t)")
  ke11/1 -> Sum84/3
  Sum85/1 -> ke10/1, ke11/1, ke12/1
  " Proces liniar26"/3(I(t)) -> k12/1
  k11/1 -> Sum83/2
  " Proces liniar26"/2(X(t)) -> k11/1
  Constant22/1 -> Sum82/1
  Sum84/1 -> " Proces liniar26"/1(" u(t)")
  ke10/1 -> Sum84/2
  ke12/1 -> Sum84/4
  Sum82/1 -> k10/1
  Sum83/1 -> Saturation29/1, Sum84/1
  " Proces liniar26"/1(" G(t)") -> Sum82/2, Sum85/2
  k12/1 -> Sum83/3
  300gg/1(" G(t)") -> Mux52/5, Scope68/1, Sum85/1
  Sum95/1 -> Saturation32/1, Sum96/1
  k16/1 -> Sum99/3
  k15/1 -> Sum99/2
  Sum99/1 -> Saturation33/1, Sum100/1
  k18/1 -> Sum87/2
  k23/1 -> Sum95/2
  k19/1 -> Sum91/1
  k21/1 -> Sum91/3
  " Proces liniar30"/2(X(t)) -> k15/1
  k22/1 -> Sum95/1
  Sum88/1 -> " Proces liniar27"/1(" u(t)")
  100g.1/1(" G(t)") -> Mux53/5, Scope70/1, Sum101/1
  Sum97/1 -> ke22/1, ke23/1, ke24/1
  ke14/1 -> Sum100/2
  k14/1 -> Sum99/1
  Sum98/1 -> k14/1
  Sum87/1 -> Saturation30/1, Sum88/1
  k20/1 -> Sum91/2
  k24/1 -> Sum95/3
  Sum89/1 -> ke13/1, ke17/1, ke18/1
  " Proces liniar30"/1(" G(t)") -> Sum98/2, Sum101/2
  Mux53/1 -> Scope69/1
  Saturation30/1 -> 10g.1/1(" u(t)")
  Sum100/1 -> " Proces liniar30"/1(" u(t)")
  ke18/1 -> Sum88/4
  Constant28/1 -> Sum98/1
  " Proces liniar30"/3(I(t)) -> k16/1
  ke24/1 -> Sum96/4
  ke15/1 -> Sum100/3
  " Proces liniar28"/2(X(t)) -> k20/1
  Sum94/1 -> k22/1
  ke16/1 -> Sum100/4
  Sum101/1 -> ke14/1, ke15/1, ke16/1
  " Proces liniar29"/1(" G(t)") -> Sum94/2, Sum97/2
  k17/1 -> Sum87/3
  Saturation33/1 -> 100g.1/1(" u(t)")
  Constant21/1 -> Mux53/2
  Sum91/1 -> Saturation31/1, Sum92/1
  Constant26/1 -> Sum90/1
  Sum96/1 -> " Proces liniar29"/1(" u(t)")
  " Proces liniar27"/3(I(t)) -> k18/1
  " Proces liniar29"/3(I(t)) -> k24/1
  " Proces liniar29"/2(X(t)) -> k23/1
  Constant27/1 -> Sum94/1
  ke23/1 -> Sum96/3
  ke17/1 -> Sum88/3
  Sum92/1 -> " Proces liniar28"/1(" u(t)")
  Sum86/1 -> k13/1
  10g.1/1(" G(t)") -> Mux53/1, Sum89/1
  " Proces liniar27"/1(" G(t)") -> Sum86/2, Sum89/2
  Saturation32/1 -> 70g.1/1(" u(t)")
  Sum90/1 -> k19/1
  70g.1/1(" G(t)") -> Mux53/4, Sum97/1
  ke22/1 -> Sum96/2
  ke20/1 -> Sum92/3
  " Proces liniar28"/1(" G(t)") -> Sum90/2, Sum93/2
  40g.1/1(" G(t)") -> Mux53/3, Sum93/1
  ke21/1 -> Sum92/4
  k13/1 -> Sum87/1
  ke13/1 -> Sum88/2
  ke19/1 -> Sum92/2
  Constant18/1 -> Sum86/1
  " Proces liniar28"/3(I(t)) -> k21/1
  Saturation31/1 -> 40g.1/1(" u(t)")
  Sum93/1 -> ke19/1, ke20/1, ke21/1
  " Proces liniar27"/2(X(t)) -> k17/1
  perturbatie8/1(p(t)) -> 10g.1/2(p(t))
  perturbatie10/1(p(t)) -> 40g.1/2(p(t))
  perturbatie12/1(p(t)) -> 70g.1/2(p(t))
  perturbatie13/1(p(t)) -> 100g.1/2(p(t))
  Sum104/1 -> K10/1
  Sum105/1 -> 40.1g1/2(u(t))
  70.1g1/2(X(t)) -> K17/1
  K15/1 -> Sum105/2
  Saturation35/1 -> Sum103/1
  Sum102/1 -> K12/1
  K13/1 -> Saturation37/1
  K19/1 -> Sum105/3
  K21/1 -> Sum109/3
  Constant31/1 -> Sum108/1
  K17/1 -> Sum107/2
  10.1g1/1(G(t)) -> Sum102/2, Scope72/2, Scope73/1
  K10/1 -> Saturation34/1
  Val. optima1/1 -> Scope72/1
  K12/1 -> Saturation35/1
  Saturation36/1 -> Sum107/1
  Sum108/1 -> K13/1
  K20/1 -> Sum107/3
  Saturation37/1 -> Sum109/1
  K11/1 -> Saturation36/1
  Sum103/1 -> 10.1g1/2(u(t))
  40.1g1/1(G(t)) -> Scope72/3, Scope74/1, Sum104/2
  K18/1 -> Sum109/2
  40.1g1/3(I(t)) -> K19/1
  Sum109/1 -> " 100.1g1"/2(u(t))
  40.1g1/2(X(t)) -> K15/1
  10.1g1/3(I(t)) -> K16/1
  Constant32/1 -> Sum102/1
  K16/1 -> Sum103/3
  70.1g1/1(G(t)) -> Scope72/4, Scope75/1, Sum106/2
  Constant30/1 -> Sum106/1
  " 100.1g1"/1(G(t)) -> Scope76/1, Scope72/5, Sum108/2
  70.1g1/3(I(t)) -> K20/1
  K14/1 -> Sum103/2
  Sum106/1 -> K11/1
  " 100.1g1"/2(X(t)) -> K18/1
  " 100.1g1"/3(I(t)) -> K21/1
  Constant29/1 -> Sum104/1
  Saturation34/1 -> Sum105/1
  10.1g1/2(X(t)) -> K14/1
  Sum107/1 -> 70.1g1/2(u(t))

== system final_model/  G0 = 200 ==
  " u(t)" : Inport
  p(t) : Inport  Port=2
  Constant : Constant  Value=p1*Gb
  Constant1 : Constant  Value=p1
  Gain : Gain  Gain=1/V
  Gain1 : Gain  Gain=n
  Gain2 : Gain  Gain=p3
  Gain3 : Gain  Gain=-p2
  Gain4 : Gain  Gain=1/V
  Integrator : Integrator
  Integrator1 : Integrator
  Integrator2 : Integrator  InitialCondition=G0
  Product : Product
  Sum : Sum  Inputs=|+-
  Sum1 : Sum  Inputs=|++
  Sum2 : Sum  Inputs=|++-
  Sum3 : Sum  Inputs=|++
  " G(t)" : Outport
  X(t) : Outport  Port=2
  I(t) : Outport  Port=3
  wires:
  " u(t)"/1 -> Gain/1
  Gain/1 -> Sum/1
  Sum/1 -> Integrator/1
  Integrator/1 -> Gain2/1, I(t)/1, Gain1/1
  Gain1/1 -> Sum/2
  Gain2/1 -> Sum1/1
  Gain3/1 -> Sum1/2
  Integrator1/1 -> Gain3/1, Sum3/2, X(t)/1
  p(t)/1 -> Gain4/1
  Gain4/1 -> Sum2/1
  Constant/1 -> Sum2/2
  Constant1/1 -> Sum3/1
  Sum2/1 -> Integrator2/1
  Product/1 -> Sum2/3
  Sum3/1 -> Product/2
  Integrator2/1 -> Product/1, " G(t)"/1
  Sum1/1 -> Integrator1/1

== system final_model/  G0 = 4 ==
  " u(t)" : Inport
  p(t) : Inport  Port=2
  Constant : Constant  Value=p1*Gb
  Constant1 : Constant  Value=p1
  Gain : Gain  Gain=1/V
  Gain1 : Gain  Gain=n
  Gain2 : Gain  Gain=p3
  Gain3 : Gain  Gain=-p2
  Gain4 : Gain  Gain=1/V
  Integrator : Integrator
  Integrator1 : Integrator
  Integrator2 : Integrator  InitialCondition=G0
  Product : Product
  Sum : Sum  Inputs=|+-
  Sum1 : Sum  Inputs=|++
  Sum2 : Sum  Inputs=|++-
  Sum3 : Sum  Inputs=|++
  " G(t)" : Outport
  X(t) : Outport  Port=2
  I(t) : Outport  Port=3
  wires:
  " u(t)"/1 -> Gain/1
  Gain/1 -> Sum/1
  Sum/1 -> Integrator/1
  Integrator/1 -> Gain2/1, I(t)/1, Gain1/1
  Gain1/1 -> Sum/2
  Gain2/1 -> Sum1/1
  Gain3/1 -> Sum1/2
  Integrator1/1 -> Gain3/1, Sum3/2, X(t)/1
  p(t)/1 -> Gain4/1
  Gain4/1 -> Sum2/1
  Constant/1 -> Sum2/2
  Constant1/1 -> Sum3/1
  Sum2/1 -> Integrator2/1
  Product/1 -> Sum2/3
  Sum3/1 -> Product/2
  Integrator2/1 -> Product/1, " G(t)"/1
  Sum1/1 -> Integrator1/1

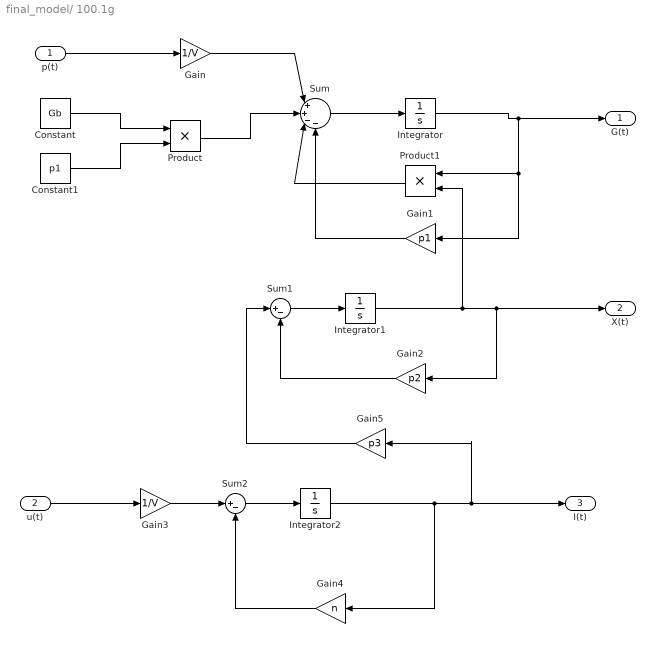
== system final_model/ 100.1g ==
  p(t) : Inport
  u(t) : Inport  Port=2
  Constant : Constant  Value=Gb
  Constant1 : Constant  Value=p1
  Gain : Gain  Gain=1/V
  Gain1 : Gain  Gain=p1
  Gain2 : Gain  Gain=p2
  Gain3 : Gain  Gain=1/V
  Gain4 : Gain  Gain=n
  Gain5 : Gain  Gain=p3
  Integrator : Integrator  InitialCondition=G0
  Integrator1 : Integrator
  Integrator2 : Integrator
  Product : Product
  Product1 : Product
  Sum : Sum  Inputs=|++--
  Sum1 : Sum  Inputs=|+-
  Sum2 : Sum  Inputs=|+-
  G(t) : Outport
  X(t) : Outport  Port=2
  I(t) : Outport  Port=3
  wires:
  Sum2/1 -> Integrator2/1
  Gain3/1 -> Sum2/1
  Sum1/1 -> Integrator1/1
  Integrator2/1 -> Gain4/1, I(t)/1, Gain5/1
  u(t)/1 -> Gain3/1
  Integrator1/1 -> Product1/2, X(t)/1, Gain2/1
  Product/1 -> Sum/2
  Integrator/1 -> G(t)/1, Gain1/1, Product1/1
  Gain5/1 -> Sum1/1
  Sum/1 -> Integrator/1
  Constant1/1 -> Product/2
  Constant/1 -> Product/1
  Gain4/1 -> Sum2/2
  Gain2/1 -> Sum1/2
  Product1/1 -> Sum/3
  Gain1/1 -> Sum/4
  p(t)/1 -> Gain/1
  Gain/1 -> Sum/1

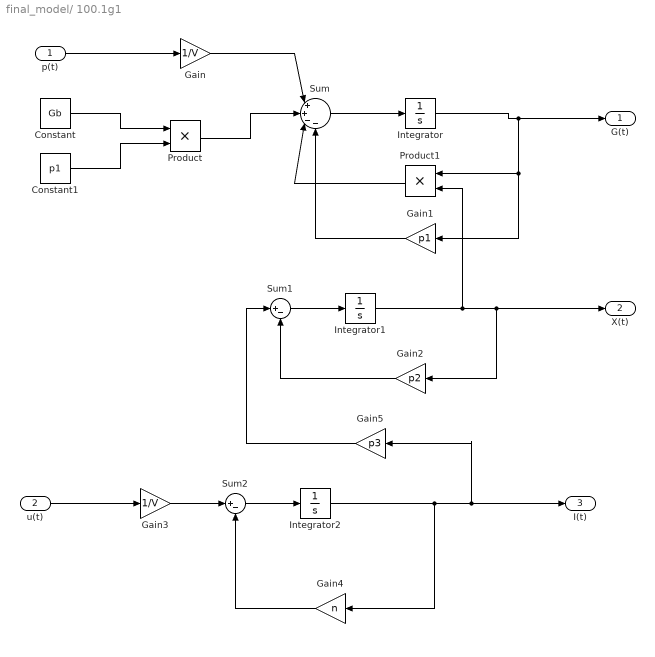
== system final_model/ 100.1g1 ==
  p(t) : Inport
  u(t) : Inport  Port=2
  Constant : Constant  Value=Gb
  Constant1 : Constant  Value=p1
  Gain : Gain  Gain=1/V
  Gain1 : Gain  Gain=p1
  Gain2 : Gain  Gain=p2
  Gain3 : Gain  Gain=1/V
  Gain4 : Gain  Gain=n
  Gain5 : Gain  Gain=p3
  Integrator : Integrator  InitialCondition=G0
  Integrator1 : Integrator
  Integrator2 : Integrator
  Product : Product
  Product1 : Product
  Sum : Sum  Inputs=|++--
  Sum1 : Sum  Inputs=|+-
  Sum2 : Sum  Inputs=|+-
  G(t) : Outport
  X(t) : Outport  Port=2
  I(t) : Outport  Port=3
  wires:
  Sum2/1 -> Integrator2/1
  Gain3/1 -> Sum2/1
  Sum1/1 -> Integrator1/1
  Integrator2/1 -> Gain4/1, I(t)/1, Gain5/1
  u(t)/1 -> Gain3/1
  Integrator1/1 -> Product1/2, X(t)/1, Gain2/1
  Product/1 -> Sum/2
  Integrator/1 -> G(t)/1, Gain1/1, Product1/1
  Gain5/1 -> Sum1/1
  Sum/1 -> Integrator/1
  Constant1/1 -> Product/2
  Constant/1 -> Product/1
  Gain4/1 -> Sum2/2
  Gain2/1 -> Sum1/2
  Product1/1 -> Sum/3
  Gain1/1 -> Sum/4
  p(t)/1 -> Gain/1
  Gain/1 -> Sum/1

== system final_model/ G0 = 10 ==
  " u(t)" : Inport
  p(t) : Inport  Port=2
  Constant : Constant  Value=p1*Gb
  Constant1 : Constant  Value=p1
  Gain : Gain  Gain=1/V
  Gain1 : Gain  Gain=n
  Gain2 : Gain  Gain=p3
  Gain3 : Gain  Gain=-p2
  Gain4 : Gain  Gain=1/V
  Integrator : Integrator
  Integrator1 : Integrator
  Integrator2 : Integrator  InitialCondition=G0
  Product : Product
  Sum : Sum  Inputs=|+-
  Sum1 : Sum  Inputs=|++
  Sum2 : Sum  Inputs=|++-
  Sum3 : Sum  Inputs=|++
  " G(t)" : Outport
  X(t) : Outport  Port=2
  I(t) : Outport  Port=3
  wires:
  " u(t)"/1 -> Gain/1
  Gain/1 -> Sum/1
  Sum/1 -> Integrator/1
  Integrator/1 -> Gain2/1, I(t)/1, Gain1/1
  Gain1/1 -> Sum/2
  Gain2/1 -> Sum1/1
  Gain3/1 -> Sum1/2
  Integrator1/1 -> Gain3/1, Sum3/2, X(t)/1
  p(t)/1 -> Gain4/1
  Gain4/1 -> Sum2/1
  Constant/1 -> Sum2/2
  Constant1/1 -> Sum3/1
  Sum2/1 -> Integrator2/1
  Product/1 -> Sum2/3
  Sum3/1 -> Product/2
  Integrator2/1 -> Product/1, " G(t)"/1
  Sum1/1 -> Integrator1/1

== system final_model/ G0 = 11 ==
  " u(t)" : Inport
  p(t) : Inport  Port=2
  Constant : Constant  Value=p1*Gb
  Constant1 : Constant  Value=p1
  Gain : Gain  Gain=1/V
  Gain1 : Gain  Gain=n
  Gain2 : Gain  Gain=p3
  Gain3 : Gain  Gain=-p2
  Gain4 : Gain  Gain=1/V
  Integrator : Integrator
  Integrator1 : Integrator
  Integrator2 : Integrator  InitialCondition=G0
  Product : Product
  Sum : Sum  Inputs=|+-
  Sum1 : Sum  Inputs=|++
  Sum2 : Sum  Inputs=|++-
  Sum3 : Sum  Inputs=|++
  " G(t)" : Outport
  X(t) : Outport  Port=2
  I(t) : Outport  Port=3
  wires:
  " u(t)"/1 -> Gain/1
  Gain/1 -> Sum/1
  Sum/1 -> Integrator/1
  Integrator/1 -> Gain2/1, I(t)/1, Gain1/1
  Gain1/1 -> Sum/2
  Gain2/1 -> Sum1/1
  Gain3/1 -> Sum1/2
  Integrator1/1 -> Gain3/1, Sum3/2, X(t)/1
  p(t)/1 -> Gain4/1
  Gain4/1 -> Sum2/1
  Constant/1 -> Sum2/2
  Constant1/1 -> Sum3/1
  Sum2/1 -> Integrator2/1
  Product/1 -> Sum2/3
  Sum3/1 -> Product/2
  Integrator2/1 -> Product/1, " G(t)"/1
  Sum1/1 -> Integrator1/1

== system final_model/ G0 = 12 ==
  " u(t)" : Inport
  p(t) : Inport  Port=2
  Constant : Constant  Value=p1*Gb
  Constant1 : Constant  Value=p1
  Gain : Gain  Gain=1/V
  Gain1 : Gain  Gain=n
  Gain2 : Gain  Gain=p3
  Gain3 : Gain  Gain=-p2
  Gain4 : Gain  Gain=1/V
  Integrator : Integrator
  Integrator1 : Integrator
  Integrator2 : Integrator  InitialCondition=G0
  Product : Product
  Sum : Sum  Inputs=|+-
  Sum1 : Sum  Inputs=|++
  Sum2 : Sum  Inputs=|++-
  Sum3 : Sum  Inputs=|++
  " G(t)" : Outport
  X(t) : Outport  Port=2
  I(t) : Outport  Port=3
  wires:
  " u(t)"/1 -> Gain/1
  Gain/1 -> Sum/1
  Sum/1 -> Integrator/1
  Integrator/1 -> Gain2/1, I(t)/1, Gain1/1
  Gain1/1 -> Sum/2
  Gain2/1 -> Sum1/1
  Gain3/1 -> Sum1/2
  Integrator1/1 -> Gain3/1, Sum3/2, X(t)/1
  p(t)/1 -> Gain4/1
  Gain4/1 -> Sum2/1
  Constant/1 -> Sum2/2
  Constant1/1 -> Sum3/1
  Sum2/1 -> Integrator2/1
  Product/1 -> Sum2/3
  Sum3/1 -> Product/2
  Integrator2/1 -> Product/1, " G(t)"/1
  Sum1/1 -> Integrator1/1

== system final_model/ G0 = 150 ==
  " u(t)" : Inport
  p(t) : Inport  Port=2
  Constant : Constant  Value=p1*Gb
  Constant1 : Constant  Value=p1
  Gain : Gain  Gain=1/V
  Gain1 : Gain  Gain=n
  Gain2 : Gain  Gain=p3
  Gain3 : Gain  Gain=-p2
  Gain4 : Gain  Gain=1/V
  Integrator : Integrator
  Integrator1 : Integrator
  Integrator2 : Integrator  InitialCondition=G0
  Product : Product
  Sum : Sum  Inputs=|+-
  Sum1 : Sum  Inputs=|++
  Sum2 : Sum  Inputs=|++-
  Sum3 : Sum  Inputs=|++
  " G(t)" : Outport
  X(t) : Outport  Port=2
  I(t) : Outport  Port=3
  wires:
  " u(t)"/1 -> Gain/1
  Gain/1 -> Sum/1
  Sum/1 -> Integrator/1
  Integrator/1 -> Gain2/1, I(t)/1, Gain1/1
  Gain1/1 -> Sum/2
  Gain2/1 -> Sum1/1
  Gain3/1 -> Sum1/2
  Integrator1/1 -> Gain3/1, Sum3/2, X(t)/1
  p(t)/1 -> Gain4/1
  Gain4/1 -> Sum2/1
  Constant/1 -> Sum2/2
  Constant1/1 -> Sum3/1
  Sum2/1 -> Integrator2/1
  Product/1 -> Sum2/3
  Sum3/1 -> Product/2
  Integrator2/1 -> Product/1, " G(t)"/1
  Sum1/1 -> Integrator1/1

== system final_model/ G0 = 250 ==
  " u(t)" : Inport
  p(t) : Inport  Port=2
  Constant : Constant  Value=p1*Gb
  Constant1 : Constant  Value=p1
  Gain : Gain  Gain=1/V
  Gain1 : Gain  Gain=n
  Gain2 : Gain  Gain=p3
  Gain3 : Gain  Gain=-p2
  Gain4 : Gain  Gain=1/V
  Integrator : Integrator
  Integrator1 : Integrator
  Integrator2 : Integrator  InitialCondition=G0
  Product : Product
  Sum : Sum  Inputs=|+-
  Sum1 : Sum  Inputs=|++
  Sum2 : Sum  Inputs=|++-
  Sum3 : Sum  Inputs=|++
  " G(t)" : Outport
  X(t) : Outport  Port=2
  I(t) : Outport  Port=3
  wires:
  " u(t)"/1 -> Gain/1
  Gain/1 -> Sum/1
  Sum/1 -> Integrator/1
  Integrator/1 -> Gain2/1, I(t)/1, Gain1/1
  Gain1/1 -> Sum/2
  Gain2/1 -> Sum1/1
  Gain3/1 -> Sum1/2
  Integrator1/1 -> Gain3/1, Sum3/2, X(t)/1
  p(t)/1 -> Gain4/1
  Gain4/1 -> Sum2/1
  Constant/1 -> Sum2/2
  Constant1/1 -> Sum3/1
  Sum2/1 -> Integrator2/1
  Product/1 -> Sum2/3
  Sum3/1 -> Product/2
  Integrator2/1 -> Product/1, " G(t)"/1
  Sum1/1 -> Integrator1/1

== system final_model/ G0 = 300 ==
  " u(t)" : Inport
  p(t) : Inport  Port=2
  Constant : Constant  Value=p1*Gb
  Constant1 : Constant  Value=p1
  Gain : Gain  Gain=1/V
  Gain1 : Gain  Gain=n
  Gain2 : Gain  Gain=p3
  Gain3 : Gain  Gain=-p2
  Gain4 : Gain  Gain=1/V
  Integrator : Integrator
  Integrator1 : Integrator
  Integrator2 : Integrator  InitialCondition=G0
  Product : Product
  Sum : Sum  Inputs=|+-
  Sum1 : Sum  Inputs=|++
  Sum2 : Sum  Inputs=|++-
  Sum3 : Sum  Inputs=|++
  " G(t)" : Outport
  X(t) : Outport  Port=2
  I(t) : Outport  Port=3
  wires:
  " u(t)"/1 -> Gain/1
  Gain/1 -> Sum/1
  Sum/1 -> Integrator/1
  Integrator/1 -> Gain2/1, I(t)/1, Gain1/1
  Gain1/1 -> Sum/2
  Gain2/1 -> Sum1/1
  Gain3/1 -> Sum1/2
  Integrator1/1 -> Gain3/1, Sum3/2, X(t)/1
  p(t)/1 -> Gain4/1
  Gain4/1 -> Sum2/1
  Constant/1 -> Sum2/2
  Constant1/1 -> Sum3/1
  Sum2/1 -> Integrator2/1
  Product/1 -> Sum2/3
  Sum3/1 -> Product/2
  Integrator2/1 -> Product/1, " G(t)"/1
  Sum1/1 -> Integrator1/1

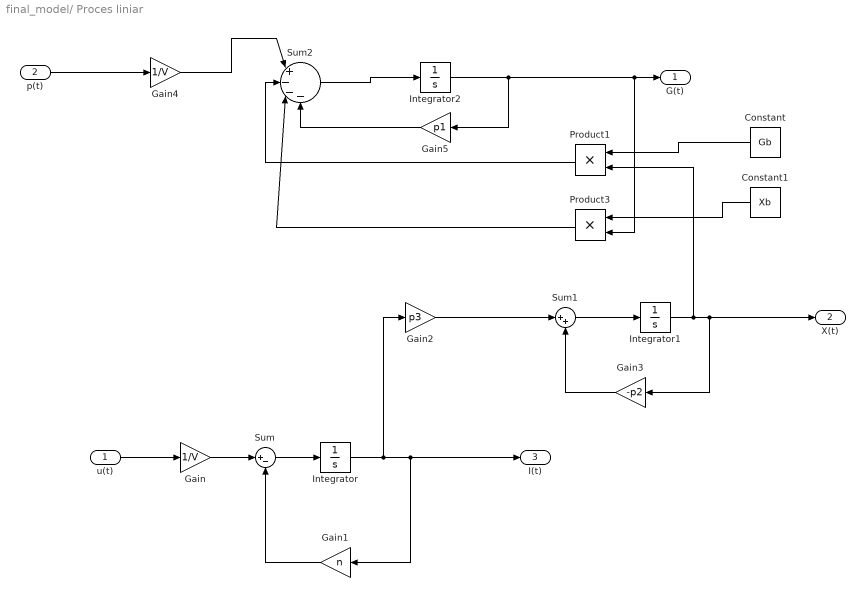
== system final_model/ Proces liniar ==
  " u(t)" : Inport
  p(t) : Inport  Port=2
  Constant : Constant  Value=Gb
  Constant1 : Constant  Value=Xb
  Gain : Gain  Gain=1/V
  Gain1 : Gain  Gain=n
  Gain2 : Gain  Gain=p3
  Gain3 : Gain  Gain=-p2
  Gain4 : Gain  Gain=1/V
  Gain5 : Gain  Gain=p1
  Integrator : Integrator
  Integrator1 : Integrator
  Integrator2 : Integrator  InitialCondition=G0
  Product1 : Product
  Product3 : Product
  Sum : Sum  Inputs=|+-
  Sum1 : Sum  Inputs=|++
  Sum2 : Sum  Inputs=|+---
  " G(t)" : Outport
  X(t) : Outport  Port=2
  I(t) : Outport  Port=3
  wires:
  Gain2/1 -> Sum1/1
  Gain/1 -> Sum/1
  " u(t)"/1 -> Gain/1
  Sum/1 -> Integrator/1
  Gain1/1 -> Sum/2
  Integrator2/1 -> Product3/2, " G(t)"/1, Gain5/1
  Integrator1/1 -> Product1/2, Gain3/1, X(t)/1
  Integrator/1 -> Gain2/1, I(t)/1, Gain1/1
  Gain3/1 -> Sum1/2
  Gain4/1 -> Sum2/1
  Gain5/1 -> Sum2/4
  p(t)/1 -> Gain4/1
  Sum1/1 -> Integrator1/1
  Sum2/1 -> Integrator2/1
  Constant/1 -> Product1/1
  Constant1/1 -> Product3/1
  Product3/1 -> Sum2/3
  Product1/1 -> Sum2/2

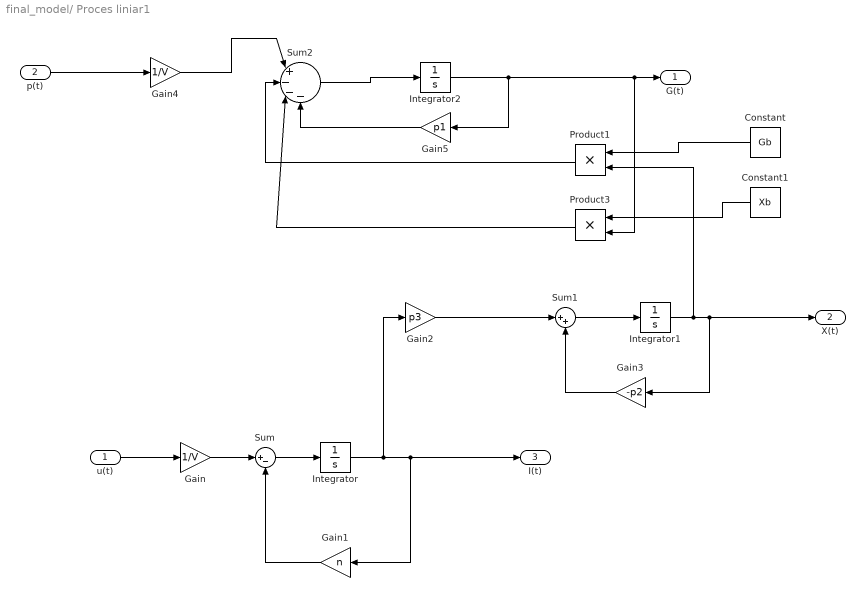
== system final_model/ Proces liniar1 ==
  " u(t)" : Inport
  p(t) : Inport  Port=2
  Constant : Constant  Value=Gb
  Constant1 : Constant  Value=Xb
  Gain : Gain  Gain=1/V
  Gain1 : Gain  Gain=n
  Gain2 : Gain  Gain=p3
  Gain3 : Gain  Gain=-p2
  Gain4 : Gain  Gain=1/V
  Gain5 : Gain  Gain=p1
  Integrator : Integrator
  Integrator1 : Integrator
  Integrator2 : Integrator  InitialCondition=G0
  Product1 : Product
  Product3 : Product
  Sum : Sum  Inputs=|+-
  Sum1 : Sum  Inputs=|++
  Sum2 : Sum  Inputs=|+---
  " G(t)" : Outport
  X(t) : Outport  Port=2
  I(t) : Outport  Port=3
  wires:
  Gain2/1 -> Sum1/1
  Gain/1 -> Sum/1
  " u(t)"/1 -> Gain/1
  Sum/1 -> Integrator/1
  Gain1/1 -> Sum/2
  Integrator2/1 -> Product3/2, " G(t)"/1, Gain5/1
  Integrator1/1 -> Product1/2, Gain3/1, X(t)/1
  Integrator/1 -> Gain2/1, I(t)/1, Gain1/1
  Gain3/1 -> Sum1/2
  Gain4/1 -> Sum2/1
  Gain5/1 -> Sum2/4
  p(t)/1 -> Gain4/1
  Sum1/1 -> Integrator1/1
  Sum2/1 -> Integrator2/1
  Constant/1 -> Product1/1
  Constant1/1 -> Product3/1
  Product3/1 -> Sum2/3
  Product1/1 -> Sum2/2

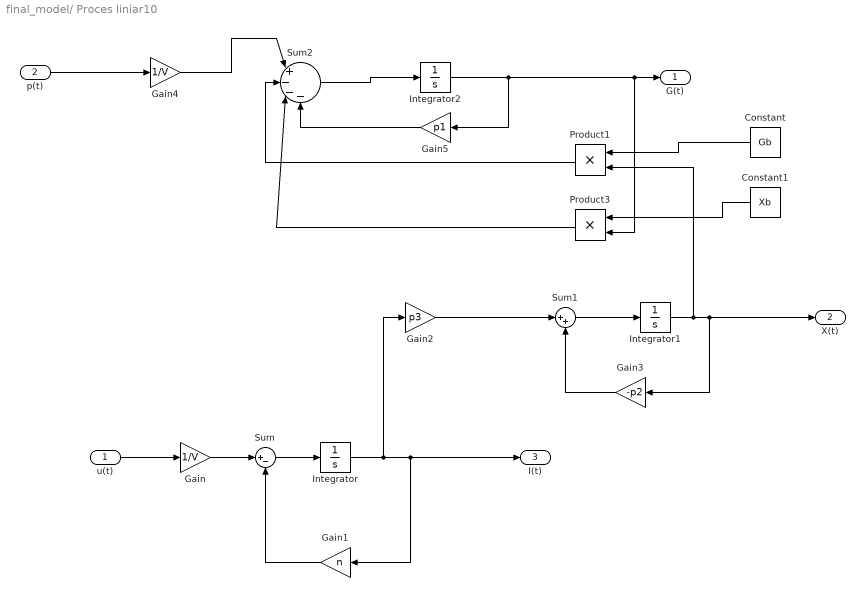
== system final_model/ Proces liniar10 ==
  " u(t)" : Inport
  p(t) : Inport  Port=2
  Constant : Constant  Value=Gb
  Constant1 : Constant  Value=Xb
  Gain : Gain  Gain=1/V
  Gain1 : Gain  Gain=n
  Gain2 : Gain  Gain=p3
  Gain3 : Gain  Gain=-p2
  Gain4 : Gain  Gain=1/V
  Gain5 : Gain  Gain=p1
  Integrator : Integrator
  Integrator1 : Integrator
  Integrator2 : Integrator  InitialCondition=G0
  Product1 : Product
  Product3 : Product
  Sum : Sum  Inputs=|+-
  Sum1 : Sum  Inputs=|++
  Sum2 : Sum  Inputs=|+---
  " G(t)" : Outport
  X(t) : Outport  Port=2
  I(t) : Outport  Port=3
  wires:
  Gain2/1 -> Sum1/1
  Gain/1 -> Sum/1
  " u(t)"/1 -> Gain/1
  Sum/1 -> Integrator/1
  Gain1/1 -> Sum/2
  Integrator2/1 -> Product3/2, " G(t)"/1, Gain5/1
  Integrator1/1 -> Product1/2, Gain3/1, X(t)/1
  Integrator/1 -> Gain2/1, I(t)/1, Gain1/1
  Gain3/1 -> Sum1/2
  Gain4/1 -> Sum2/1
  Gain5/1 -> Sum2/4
  p(t)/1 -> Gain4/1
  Sum1/1 -> Integrator1/1
  Sum2/1 -> Integrator2/1
  Constant/1 -> Product1/1
  Constant1/1 -> Product3/1
  Product3/1 -> Sum2/3
  Product1/1 -> Sum2/2

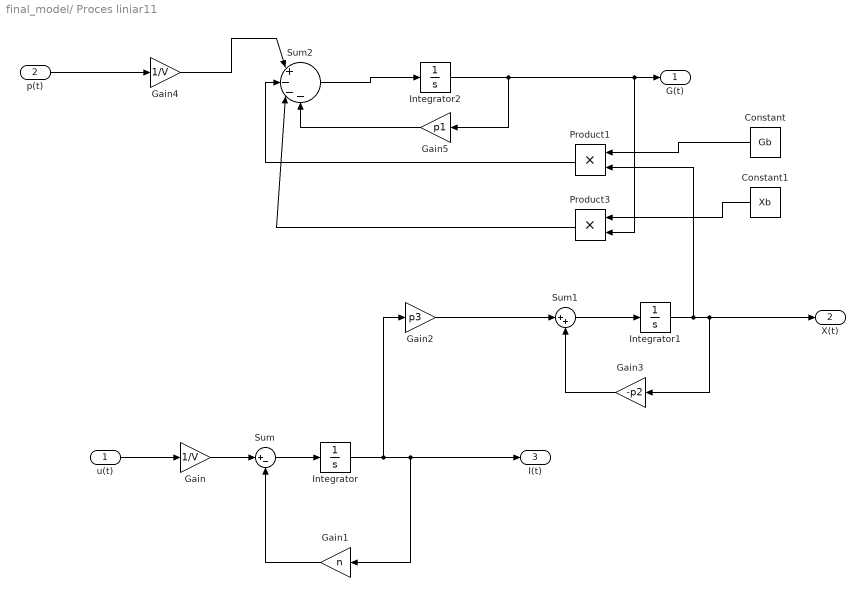
== system final_model/ Proces liniar11 ==
  " u(t)" : Inport
  p(t) : Inport  Port=2
  Constant : Constant  Value=Gb
  Constant1 : Constant  Value=Xb
  Gain : Gain  Gain=1/V
  Gain1 : Gain  Gain=n
  Gain2 : Gain  Gain=p3
  Gain3 : Gain  Gain=-p2
  Gain4 : Gain  Gain=1/V
  Gain5 : Gain  Gain=p1
  Integrator : Integrator
  Integrator1 : Integrator
  Integrator2 : Integrator  InitialCondition=G0
  Product1 : Product
  Product3 : Product
  Sum : Sum  Inputs=|+-
  Sum1 : Sum  Inputs=|++
  Sum2 : Sum  Inputs=|+---
  " G(t)" : Outport
  X(t) : Outport  Port=2
  I(t) : Outport  Port=3
  wires:
  Gain2/1 -> Sum1/1
  Gain/1 -> Sum/1
  " u(t)"/1 -> Gain/1
  Sum/1 -> Integrator/1
  Gain1/1 -> Sum/2
  Integrator2/1 -> Product3/2, " G(t)"/1, Gain5/1
  Integrator1/1 -> Product1/2, Gain3/1, X(t)/1
  Integrator/1 -> Gain2/1, I(t)/1, Gain1/1
  Gain3/1 -> Sum1/2
  Gain4/1 -> Sum2/1
  Gain5/1 -> Sum2/4
  p(t)/1 -> Gain4/1
  Sum1/1 -> Integrator1/1
  Sum2/1 -> Integrator2/1
  Constant/1 -> Product1/1
  Constant1/1 -> Product3/1
  Product3/1 -> Sum2/3
  Product1/1 -> Sum2/2
